simulink model "altitudeCheck"  (R2018b)
settings: Solver=VariableStepAuto  StartTime=0.0  StopTime=200  RelTol=1e-3
values from neighbouring files (symbols this model uses):
  plane = AirPlane("NT-33A_4.xlsx")    [entryPoint.m]    (also in main.m)
  servo = tf(10,[1 10])    [main.m]
libraries: cstblocks x4, simulink_extras x3
settings Model: Creator=Mo.Hatem  LastModifiedBy=OWNER

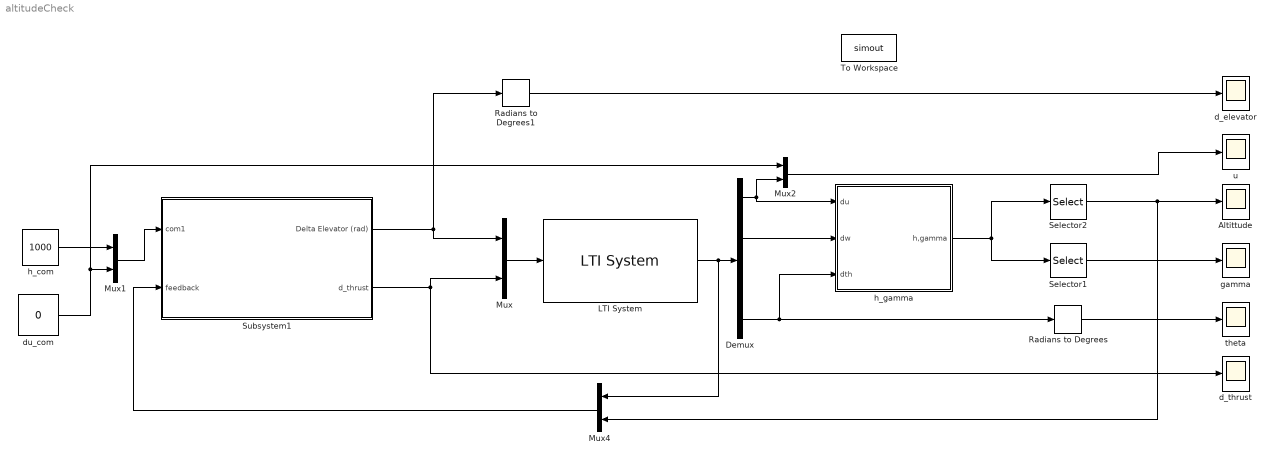
== system altitudeCheck ==
  Altittude : Scope
  Demux : Demux
  LTI System : cstblocks/LTI System  sys=LongSS  IC=[]
  Mux{,1..2,4} (4 alike) : Mux  Inputs=2
  Radians to Degrees : simulink_extras/Transformations/Radians to Degrees
  Radians to Degrees1 : simulink_extras/Transformations/Radians to Degrees
  Selector1 : Selector  InputPortWidth=2  IndexOptions=Index vector (dialog)  Indices=[2]  OutputSizes=1
  Selector2 : Selector  InputPortWidth=2  IndexOptions=Index vector (dialog)  Indices=[1]  OutputSizes=1
  Subsystem1 : Subsystem
  To Workspace : ToWorkspace  VariableName=simout  SaveFormat=Timeseries  SampleTime=-1
  d_elevator : Scope
  d_thrust : Scope
  du_com : Constant  Value=0
  gamma : Scope
  h_com : Constant  Value=1000
  h_gamma : Subsystem
  theta : Scope
  u : Scope
  wires:
  Mux/1 -> LTI System/1
  LTI System/1 -> Mux4/1, Demux/1
  Demux/4 -> h_gamma/3(dth), Radians to Degrees/1
  Demux/2 -> h_gamma/2(dw)
  h_gamma/1(h,gamma) -> Selector2/1, Selector1/1
  Selector1/1 -> gamma/1
  Demux/1 -> h_gamma/1(du), Mux2/2
  Mux1/1 -> Subsystem1/1(com1)
  Selector2/1 -> Mux4/2, Altittude/1
  Mux2/1 -> u/1
  du_com/1 -> Mux2/1, Mux1/2
  Subsystem1/1(Delta Elevator (rad)) -> Radians to Degrees1/1, Mux/1
  Radians to Degrees1/1 -> d_elevator/1
  h_com/1 -> Mux1/1
  Mux4/1 -> Subsystem1/2(feedback)
  Radians to Degrees/1 -> theta/1
  Subsystem1/2(d_thrust) -> Mux/2, d_thrust/1

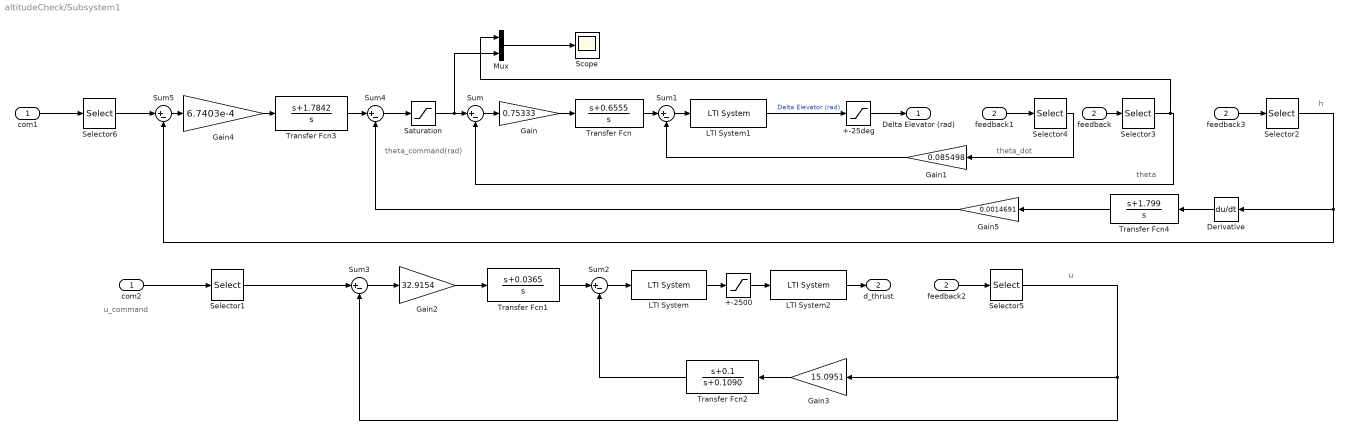
== system altitudeCheck/Subsystem1 ==
  note: u_command
  note: u
  note: theta
  note: theta_command(rad)
  note: theta_dot
  note: h
  com1 : Inport
  feedback : Inport  Port=2
  +-2500 : Saturate  UpperLimit=2500  LowerLimit=-2500
  +-25deg : Saturate  UpperLimit=25*pi/180  LowerLimit=-25*pi/180
  Derivative : Derivative
  Gain : Gain  Gain=0.75333
  Gain1 : Gain  Gain=0.085498
  Gain2 : Gain  Gain=32.9154
  Gain3 : Gain  Gain=15.0951
  Gain4 : Gain  Gain=6.7403e-4
  Gain5 : Gain  Gain=0.0014691
  LTI System : cstblocks/LTI System  sys=servo  IC=[]
  LTI System1 : cstblocks/LTI System  sys=-servo  IC=[]
  LTI System2 : cstblocks/LTI System  sys=engine_timelag  IC=[]
  Mux : Mux  Inputs=2
  Saturation : Saturate  LowerLimit=-.5
  Scope : Scope
  Selector1 : Selector  InputPortWidth=2  IndexOptions=Index vector (dialog)  Indices=[2]  OutputSizes=1
  Selector2 : Selector  InputPortWidth=5  IndexOptions=Index vector (dialog)  Indices=[5]  OutputSizes=1
  Selector3 : Selector  InputPortWidth=5  IndexOptions=Index vector (dialog)  Indices=[4]  OutputSizes=1
  Selector4 : Selector  InputPortWidth=5  IndexOptions=Index vector (dialog)  Indices=[3]  OutputSizes=1
  Selector5 : Selector  InputPortWidth=5  IndexOptions=Index vector (dialog)  Indices=[1]  OutputSizes=1
  Selector6 : Selector  InputPortWidth=2  IndexOptions=Index vector (dialog)  Indices=[1]  OutputSizes=1
  Sum{,1..5} (6 alike) : Sum  Inputs=|+-
  Transfer Fcn : TransferFcn  Numerator=[1 +0.6555]  Denominator=[1 0]
  Transfer Fcn1 : TransferFcn  Numerator=[1 0.0365]  Denominator=[1 0]
  Transfer Fcn2 : TransferFcn  Numerator=[1 0.1]  Denominator=[1 0.1090]
  Transfer Fcn3 : TransferFcn  Numerator=[1 1.7842]  Denominator=[1 0]
  Transfer Fcn4 : TransferFcn  Numerator=[1 +1.799]  Denominator=[1 0]
  com2 : InportShadow
  feedback1 : InportShadow  Port=2
  feedback2 : InportShadow  Port=2
  feedback3 : InportShadow  Port=2
  Delta Elevator (rad) : Outport  VectorParamsAs1DForOutWhenUnconnected=on
  d_thrust : Outport  Port=2  VectorParamsAs1DForOutWhenUnconnected=on
  wires:
  Transfer Fcn/1 -> Sum1/1
  Gain/1 -> Transfer Fcn/1
  Gain1/1 -> Sum1/2
  Sum1/1 -> LTI System1/1
  Sum/1 -> Gain/1
  LTI System1/1 -> +-25deg/1  "Delta Elevator (rad)"
  Selector3/1 -> Mux/1, Sum/2
  LTI System/1 -> +-2500/1
  Sum2/1 -> LTI System/1
  Selector5/1 -> Gain3/1, Sum3/2
  Transfer Fcn1/1 -> Sum2/1
  Gain3/1 -> Transfer Fcn2/1
  Gain2/1 -> Transfer Fcn1/1
  Transfer Fcn2/1 -> Sum2/2
  Sum3/1 -> Gain2/1
  com2/1 -> Selector1/1
  Selector1/1 -> Sum3/1
  feedback1/1 -> Selector4/1
  feedback/1 -> Selector3/1
  Selector4/1 -> Gain1/1
  LTI System2/1 -> d_thrust/1
  feedback2/1 -> Selector5/1
  Sum5/1 -> Gain4/1
  Sum4/1 -> Saturation/1
  feedback3/1 -> Selector2/1
  Selector2/1 -> Derivative/1, Sum5/2
  com1/1 -> Selector6/1
  Selector6/1 -> Sum5/1
  Gain4/1 -> Transfer Fcn3/1
  Transfer Fcn3/1 -> Sum4/1
  Gain5/1 -> Sum4/2
  Transfer Fcn4/1 -> Gain5/1
  Derivative/1 -> Transfer Fcn4/1
  Mux/1 -> Scope/1
  Saturation/1 -> Mux/2, Sum/1
  +-2500/1 -> LTI System2/1
  +-25deg/1 -> Delta Elevator (rad)/1

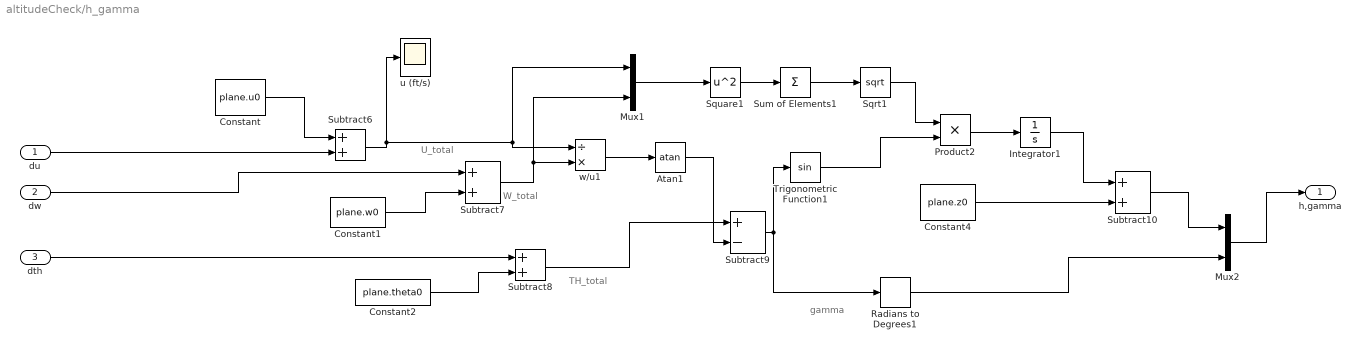
== system altitudeCheck/h_gamma ==
  note: U_total
  note: W_total
  note: TH_total
  note: gamma
  du : Inport
  dw : Inport  Port=2
  dth : Inport  Port=3
  Atan1 : Trigonometry  Operator=atan
  Constant : Constant  Value=plane.u0
  Constant1 : Constant  Value=plane.w0
  Constant2 : Constant  Value=plane.theta0  VectorParams1D=off
  Constant4 : Constant  Value=plane.z0
  Integrator1 : Integrator
  Mux1 : Mux  Inputs=2
  Mux2 : Mux  Inputs=2
  Product2 : Product
  Radians to Degrees1 : simulink_extras/Transformations/Radians to Degrees
  Sqrt1 : Sqrt  SaturateOnIntegerOverflow=on
  Square1 : Math  Operator=square  SaturateOnIntegerOverflow=on
  Subtract{6..8,10} (4 alike) : Sum
  Subtract9 : Sum  Inputs=+-
  Sum of Elements1 : Sum  Inputs=+
  Trigonometric Function1 : Trigonometry
  u (ft/s) : Scope
  w/u1 : Product  Inputs=/*
  h,gamma : Outport
  wires:
  Constant4/1 -> Subtract10/2
  w/u1/1 -> Atan1/1
  Subtract7/1 -> w/u1/2, Mux1/2
  Constant1/1 -> Subtract7/2
  Square1/1 -> Sum of Elements1/1
  Radians to Degrees1/1 -> Mux2/2
  Subtract8/1 -> Subtract9/1
  Constant/1 -> Subtract6/1
  Subtract9/1 -> Trigonometric Function1/1, Radians to Degrees1/1
  Sum of Elements1/1 -> Sqrt1/1
  Trigonometric Function1/1 -> Product2/2
  Constant2/1 -> Subtract8/2
  du/1 -> Subtract6/2
  dth/1 -> Subtract8/1
  Sqrt1/1 -> Product2/1
  dw/1 -> Subtract7/1
  Subtract6/1 -> u (ft/s)/1, w/u1/1, Mux1/1
  Integrator1/1 -> Subtract10/1
  Mux1/1 -> Square1/1
  Product2/1 -> Integrator1/1
  Atan1/1 -> Subtract9/2
  Subtract10/1 -> Mux2/1
  Mux2/1 -> h,gamma/1
